simulink model "motor_block"  (R2023b)
settings: Solver=VariableStepAuto  StartTime=0.0  StopTime=SIM_TIME  RelTol=1e-3
values from neighbouring files (symbols this model uses):
  B = 1.1e-5    (= 1.1e-05)    [load_params.m]
  J = 1.15e-6    (= 1.15e-06)    [load_params.m]
  Ke = Kt    (= 0.0799)    [load_params.m]
  Kt = 79.9e-3    (= 0.0799)    [load_params.m]
  L = 708e-6    (= 0.000708)    [load_params.m]
  MR = 6.5e-3    (= 0.0065)    [load_params.m]
  R = 2.59    [load_params.m]
  U_MAX = 12.16    [load_params.m]
  USE_OL = 1    [plot_logs.m]
settings Model: Creator=farfar  LastModifiedBy=farfar
settings DataIOCC: ReturnWorkspaceOutputsName=simu

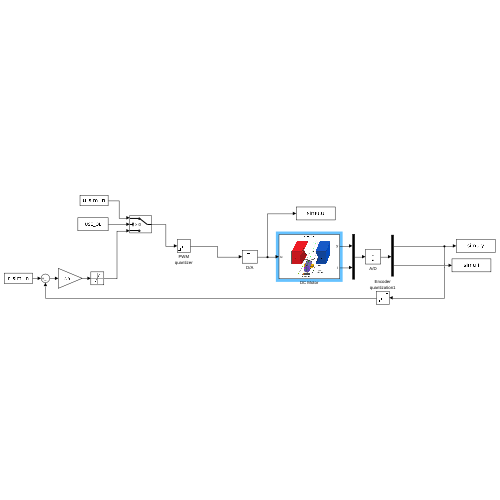
[thumbnail: Simulink's stored preview of the top-level diagram]
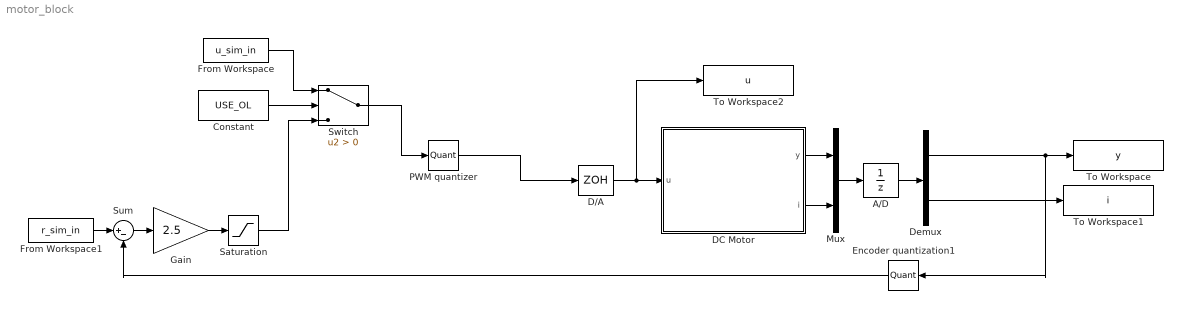
== system motor_block ==
  A/D : UnitDelay  SampleTime=1e-3  HasFrameUpgradeWarning=on
  Constant : Constant  Value=USE_OL
  D/A : ZeroOrderHold  SampleTime=1e-3
  DC Motor : Subsystem
      mask Display: image('motor.jpg');
  Demux : Demux  Outputs=2
  Encoder quantization1 : Quantizer  QuantizationInterval=2*pi/(4*5120)
  From Workspace : FromWorkspace  VariableName=u_sim_in
  From Workspace1 : FromWorkspace  VariableName=r_sim_in
  Gain : Gain  Gain=2.5
  Mux : Mux  Inputs=2
  PWM quantizer : Quantizer  QuantizationInterval=12/2^11
  Saturation : Saturate  UpperLimit=U_MAX  LowerLimit=-U_MAX
  Sum : Sum  Inputs=|+-
  Switch : Switch  Criteria=u2 > Threshold  SaturateOnIntegerOverflow=off  InputSameDT=off
  To Workspace : ToWorkspace  VariableName=y  SampleTime=1e-3
  To Workspace1 : ToWorkspace  VariableName=i  SampleTime=1e-3;
  To Workspace2 : ToWorkspace  VariableName=u  SampleTime=1e-3
  wires:
  Switch/1 -> PWM quantizer/1
  PWM quantizer/1 -> D/A/1
  Mux/1 -> A/D/1
  DC Motor/1(y) -> Mux/1
  DC Motor/2(i) -> Mux/2
  A/D/1 -> Demux/1
  Demux/2 -> To Workspace1/1
  Sum/1 -> Gain/1
  From Workspace1/1 -> Sum/1
  From Workspace/1 -> Switch/1
  Gain/1 -> Saturation/1
  Saturation/1 -> Switch/3
  Demux/1 -> Encoder quantization1/1, To Workspace/1
  D/A/1 -> To Workspace2/1, DC Motor/1(u)
  Constant/1 -> Switch/2
  Encoder quantization1/1 -> Sum/2

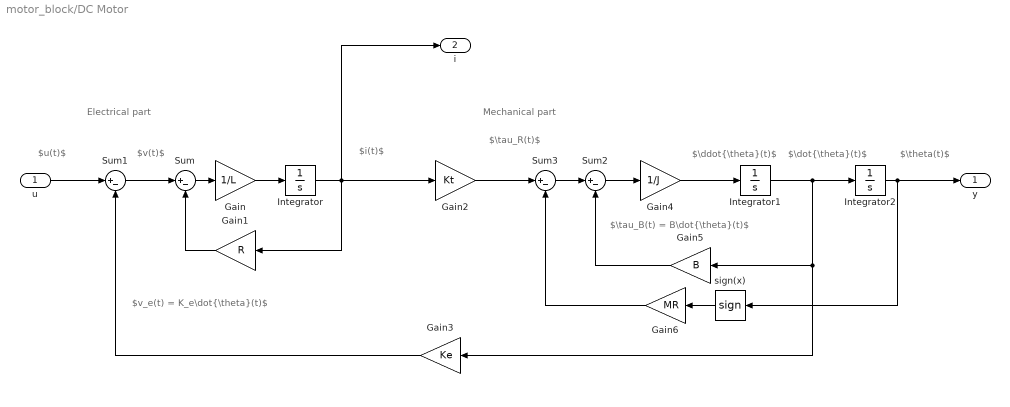
== system motor_block/DC Motor ==
  note: $v_e(t) = K_e\dot{\theta}(t)$
  note: $\theta(t)$
  note: Electrical part
  note: Mechanical part
  note: $\tau_B(t) = B\dot{\theta}(t)$
  note: $u(t)$
  note: $\dot{\theta}(t)$
  note: $\tau_R(t)$
  note: $\ddot{\theta}(t)$
  note: $i(t)$
  note: $v(t)$
  u : Inport
  Gain : Gain  Gain=1/L
  Gain1 : Gain  Gain=R
  Gain2 : Gain  Gain=Kt
  Gain3 : Gain  Gain=Ke
  Gain4 : Gain  Gain=1/J
  Gain5 : Gain  Gain=B
  Gain6 : Gain  Gain=MR
  Integrator : Integrator
  Integrator1 : Integrator
  Integrator2 : Integrator
  Sum{,1..3} (4 alike) : Sum  Inputs=|+-
  sign(x) : Signum
  y : Outport
  i : Outport  Port=2
  wires:
  Gain/1 -> Integrator/1
  Integrator2/1 -> sign(x)/1, y/1
  Gain2/1 -> Sum3/1
  Sum1/1 -> Sum/1
  Gain1/1 -> Sum/2
  Gain3/1 -> Sum1/2
  Integrator1/1 -> Gain5/1, Gain3/1, Integrator2/1
  Gain5/1 -> Sum2/2
  Integrator/1 -> i/1, Gain2/1, Gain1/1
  Sum2/1 -> Gain4/1
  Sum/1 -> Gain/1
  u/1 -> Sum1/1
  Gain4/1 -> Integrator1/1
  Sum3/1 -> Sum2/1
  sign(x)/1 -> Gain6/1
  Gain6/1 -> Sum3/2
